simulink model "Concatenate_TestGen6"  (R2017b)
settings: Solver=FixedStepDiscrete  StartTime=0.0  StopTime=10.0  RelTol=1e-3
undefined symbols (not defined in the file): Block_TestLib, enable
settings Model: Creator=ktrinh  LastModifiedBy=ktrinh
settings DebuggingCC: ParameterOverflowMsg=none

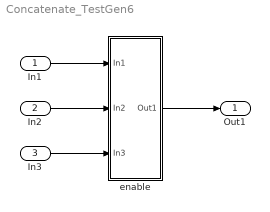
== system Concatenate_TestGen6 ==
  In1 : Inport
  In2 : Inport  Port=2
  In3 : Inport  Port=3
  enable : Subsystem  AncestorBlock=Block_TestLib/enable
  Out1 : Outport
  wires:
  In1/1 -> enable/1(In1)
  In2/1 -> enable/2(In2)
  In3/1 -> enable/3(In3)
  enable/1(Out1) -> Out1/1

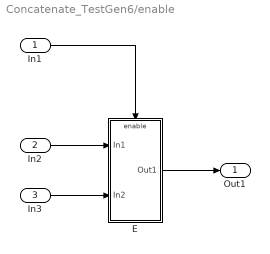
== system Concatenate_TestGen6/enable ==
  In1 : Inport  OutDataTypeStr=boolean
  In2 : Inport  Port=2
  In3 : Inport  Port=3
  E : Subsystem  TreatAsAtomicUnit=on
  Out1 : Outport
  wires:
  In1/1 -> E/Enable
  In2/1 -> E/1(In1)
  In3/1 -> E/2(In2)
  E/1(Out1) -> Out1/1

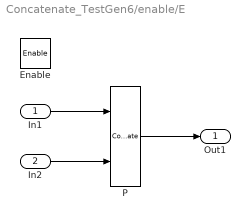
== system Concatenate_TestGen6/enable/E ==
  In1 : Inport  OutDataTypeStr=double  PortDimensions=[2 4 5]
  In2 : Inport  Port=2  OutDataTypeStr=double  PortDimensions=[2 4 5]
  Enable : EnablePort
  P : Concatenate  Mode=Multidimensional array  ConcatenateDimension=2
  Out1 : Outport
  wires:
  In1/1 -> P/1
  In2/1 -> P/2
  P/1 -> Out1/1
